simulink model "test_any"  (R2017b)
settings: Solver=FixedStepDiscrete  StartTime=0.0  StopTime=10.0  FixedStep=0.100000  RelTol=1e-3
model workspace (MAT data in the model file):
  already_pp = 1
settings Model: Creator=fconzelm  LastModifiedBy=hbourbou
settings DebuggingCC: AlgebraicLoopMsg=error  ArtificialAlgebraicLoopMsg=error  SingleTaskRateTransMsg=error

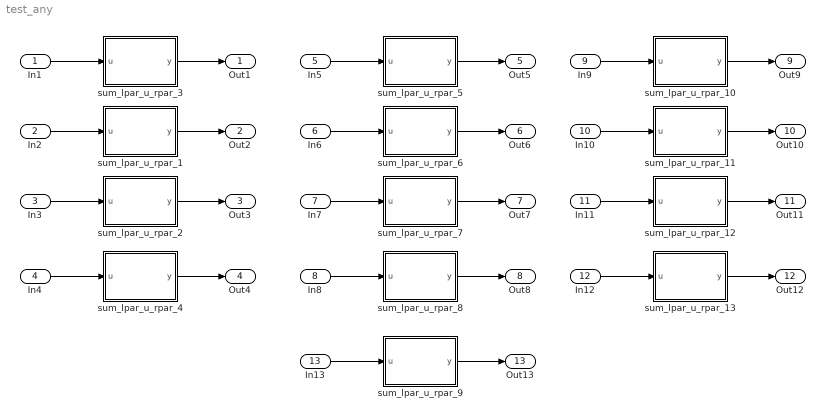
== system test_any ==
  In1 : Inport  PortDimensions=[1 3]
  In2 : Inport  Port=2  PortDimensions=[3 1]
  In3 : Inport  Port=3  PortDimensions=1
  In4 : Inport  Port=4  PortDimensions=[4 5]
  In5 : Inport  Port=5  PortDimensions=[1 3]
  In6 : Inport  Port=6  PortDimensions=[3 1]
  In7 : Inport  Port=7  PortDimensions=1
  In8 : Inport  Port=8  PortDimensions=[4 5]
  In9 : Inport  Port=9  PortDimensions=[1 3]
  In10 : Inport  Port=10  PortDimensions=[3 1]
  In11 : Inport  Port=11  PortDimensions=1
  In12 : Inport  Port=12  PortDimensions=[4 5]
  In13 : Inport  Port=13  PortDimensions=[4 5]
  sum_lpar_u_rpar_1 : MATLAB Function  TreatAsAtomicUnit=on
  sum_lpar_u_rpar_10 : MATLAB Function  TreatAsAtomicUnit=on
  sum_lpar_u_rpar_11 : MATLAB Function  TreatAsAtomicUnit=on
  sum_lpar_u_rpar_12 : MATLAB Function  TreatAsAtomicUnit=on
  sum_lpar_u_rpar_13 : MATLAB Function  TreatAsAtomicUnit=on
  sum_lpar_u_rpar_2 : MATLAB Function  TreatAsAtomicUnit=on
  sum_lpar_u_rpar_3 : MATLAB Function  TreatAsAtomicUnit=on
  sum_lpar_u_rpar_4 : MATLAB Function  TreatAsAtomicUnit=on
  sum_lpar_u_rpar_5 : MATLAB Function  TreatAsAtomicUnit=on
  sum_lpar_u_rpar_6 : MATLAB Function  TreatAsAtomicUnit=on
  sum_lpar_u_rpar_7 : MATLAB Function  TreatAsAtomicUnit=on
  sum_lpar_u_rpar_8 : MATLAB Function  TreatAsAtomicUnit=on
  sum_lpar_u_rpar_9 : MATLAB Function  TreatAsAtomicUnit=on
  Out1 : Outport
  Out2 : Outport  Port=2
  Out3 : Outport  Port=3
  Out4 : Outport  Port=4
  Out5 : Outport  Port=5
  Out6 : Outport  Port=6
  Out7 : Outport  Port=7
  Out8 : Outport  Port=8
  Out9 : Outport  Port=9
  Out10 : Outport  Port=10
  Out11 : Outport  Port=11
  Out12 : Outport  Port=12
  Out13 : Outport  Port=13
  wires:
  In1/1 -> sum_lpar_u_rpar_3/1(u)
  sum_lpar_u_rpar_3/1(y) -> Out1/1
  sum_lpar_u_rpar_1/1(y) -> Out2/1
  In2/1 -> sum_lpar_u_rpar_1/1(u)
  sum_lpar_u_rpar_2/1(y) -> Out3/1
  In3/1 -> sum_lpar_u_rpar_2/1(u)
  sum_lpar_u_rpar_4/1(y) -> Out4/1
  In4/1 -> sum_lpar_u_rpar_4/1(u)
  sum_lpar_u_rpar_5/1(y) -> Out5/1
  In5/1 -> sum_lpar_u_rpar_5/1(u)
  sum_lpar_u_rpar_6/1(y) -> Out6/1
  sum_lpar_u_rpar_7/1(y) -> Out7/1
  In6/1 -> sum_lpar_u_rpar_6/1(u)
  In7/1 -> sum_lpar_u_rpar_7/1(u)
  sum_lpar_u_rpar_8/1(y) -> Out8/1
  In8/1 -> sum_lpar_u_rpar_8/1(u)
  sum_lpar_u_rpar_10/1(y) -> Out9/1
  In9/1 -> sum_lpar_u_rpar_10/1(u)
  sum_lpar_u_rpar_11/1(y) -> Out10/1
  sum_lpar_u_rpar_12/1(y) -> Out11/1
  In10/1 -> sum_lpar_u_rpar_11/1(u)
  In11/1 -> sum_lpar_u_rpar_12/1(u)
  sum_lpar_u_rpar_13/1(y) -> Out12/1
  In12/1 -> sum_lpar_u_rpar_13/1(u)
  In13/1 -> sum_lpar_u_rpar_9/1(u)
  sum_lpar_u_rpar_9/1(y) -> Out13/1

== matlab function test_any/sum_lpar_u_rpar_1 ==
  data: u input; y output
function y = fcn(u)

y = any(u);

== matlab function test_any/sum_lpar_u_rpar_2 ==
  data: u input; y output
function y = fcn(u)

y = any(u);

== matlab function test_any/sum_lpar_u_rpar_3 ==
  data: u input; y output
function y = fcn(u)

y = any(u);

== matlab function test_any/sum_lpar_u_rpar_4 ==
  data: u input; y output
function y = fcn(u)

y = any(u);

== matlab function test_any/sum_lpar_u_rpar_5 ==
  data: u input; y output
function y = fcn(u)

y = any(u, 1);

== matlab function test_any/sum_lpar_u_rpar_6 ==
  data: u input; y output
function y = fcn(u)

y = any(u, 1);

== matlab function test_any/sum_lpar_u_rpar_7 ==
  data: u input; y output
function y = fcn(u)

y = any(u, 1);

== matlab function test_any/sum_lpar_u_rpar_8 ==
  data: u input; y output
function y = fcn(u)

y = any(u, 1);

== matlab function test_any/sum_lpar_u_rpar_9 ==
  data: u input; y output
function y = fcn(u)

y = any(any(u));

== matlab function test_any/sum_lpar_u_rpar_10 ==
  data: u input; y output
function y = fcn(u)

y = any(u, 2);

== matlab function test_any/sum_lpar_u_rpar_11 ==
  data: u input; y output
function y = fcn(u)

y = any(u, 2);

== matlab function test_any/sum_lpar_u_rpar_12 ==
  data: u input; y output
function y = fcn(u)

y = any(u, 2);

== matlab function test_any/sum_lpar_u_rpar_13 ==
  data: u input; y output
function y = fcn(u)

y = any(u, 2);
